simulink model "Longitudinal_Stability_Model"  (R2013a)
settings: Solver=ode45  StartTime=0.0  StopTime=15  RelTol=1e-6
values from neighbouring files (symbols this model uses):
  DEN = poly(p{1})    [Wrap_Flat_Earth.m]
  K = 0    [Wrap_Flat_Earth.m]
  NUM = poly(z{1})*k    [Wrap_Flat_Earth.m]
undefined symbols (not defined in the file or in its folder): sigbuilder_block
libraries: simulink_extras x1
settings Model: Creator=Willdog  LastModifiedBy=justiceb

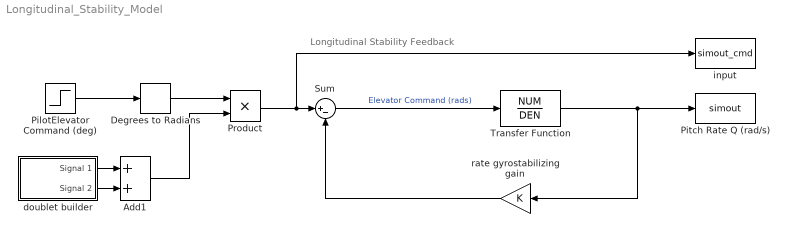
== system Longitudinal_Stability_Model ==
  note: Longitudinal Stability Feedback
  Add1 : Sum
  Degrees to Radians : simulink_extras/Transformations/Degrees to Radians
  PilotElevator Command (deg) : Step  Time=0  SampleTime=0
  Pitch Rate Q (rad/s) : ToWorkspace  VariableName=simout  SampleTime=-1  SaveFormat=Timeseries
  Product : Product
  Sum : Sum  Inputs=|+-
  Transfer Function : TransferFcn  Numerator=NUM  Denominator=DEN
  doublet builder : Subsystem  Tag=STV Subsys  LoadFcn=sigbuilder_block('load');  StartFcn=sigbuilder_block('start');  StopFcn=sigbuilder_block('stop');  ClipboardFcn=sigbuilder_block('clipboard');  mask(Sigbuilder block){}
      mask help: Sigbuilder GUI
      mask init:
      | if ~strcmp(get_param(bdroot(gcbh),'SimulationStatus'),'stopped') tuvar = sigbuilder_block('maskInit'); end
      settings: CopyFcn=sigbuilder_block('copy');  DeleteFcn=sigbuilder_block('delete');  ModelCloseFcn=sigbuilder_block('modelClose');  PreSaveFcn=sigbuilder_block('preSave');  PauseFcn=sigbuilder_block('pause')  ContinueFcn=sigbuilder_block('continue')  NameChangeFcn=sigbuilder_block('namechange');  OpenFcn=sigbuilder_block('open',[437.25 199.5 550.5 399.75 ]);  CloseFcn=sigbuilder_block('close');
      mask Display: plot(0,0,100,100,[10,10,40,40,10],[80,20,20,80,80],[40,10],[50,50], [40,27,10],[65,72,56],[40,25,25,10],[28,28,43,43]);
  input : ToWorkspace  VariableName=simout_cmd  SampleTime=-1  SaveFormat=Timeseries
  rate gyrostabilizing gain : Gain  Gain=K
  wires:
  Sum/1 -> Transfer Function/1  "Elevator Command (rads)"
  rate gyrostabilizing gain/1 -> Sum/2
  Transfer Function/1 -> rate gyrostabilizing gain/1, Pitch Rate Q (rad/s)/1
  Add1/1 -> Product/2
  doublet builder/1(Signal 1) -> Add1/1
  doublet builder/2(Signal 2) -> Add1/2
  Product/1 -> input/1, Sum/1
  PilotElevator Command (deg)/1 -> Degrees to Radians/1
  Degrees to Radians/1 -> Product/1

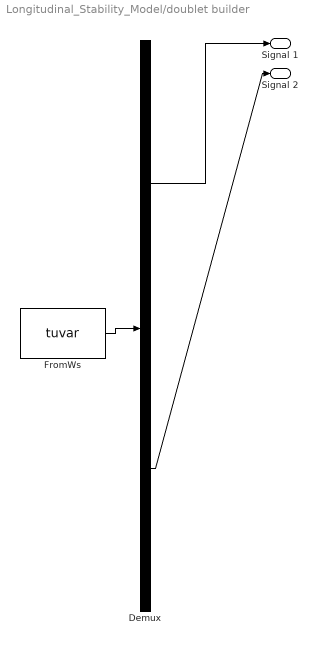
== system Longitudinal_Stability_Model/doublet builder ==
  Demux : Demux  Tag=STV Demux  Outputs=2
  FromWs : FromWorkspace  Tag=STV FromWs  VariableName=tuvar  SampleTime=0
      SigBuilderData=|
      | common.afterFinalStr = 'Extrapolate'
      | common.sampleTime = 0
      | dataSet.timeRange = [0 10]
      | dataSet.name = 'Group 1'
      | sbobj.Groups.Name = 'Group 1'
      | sbobj.Groups.Signals(1).Name = 'Signal 1'
      | sbobj.Groups.Signals(1).XData = [0 1 1 2 2 10]
      | sbobj.Groups.Signals(1).YData = [0 0 1 1 0 0]
      | sbobj.Groups.Signals(2).Name = 'Signal 2'
      | sbobj.Groups.Signals(2).XData = [0 2 2 3 3 10]
      | sbobj.Groups.Signals(2).YData = [0 0 -1 -1 0 0]
  Signal 1 : Outport  Tag=STV Outport
  Signal 2 : Outport  Tag=STV Outport  Port=2
  wires:
  Demux/1 -> Signal 1/1
  FromWs/1 -> Demux/1
  Demux/2 -> Signal 2/1
